simulink model "lazo_cerrado"  (Simulink 7.6)
settings: Solver=ode45  StartTime=0.0  StopTime=10.0  RelTol=1e-3
values from neighbouring files (symbols this model uses):
  K = [-0.22360679775 6.24198343522e-16 0.22360679775 -2.24770339741e-15 0 0 0 0 4.72115563111e-31 -4.72115563111e-31 4.72115563111e-31 -4.72115563111e-31 ... (144 elements, 12x12)]    [K.mat]
undefined symbols (not defined in the file or in its folder): g, Ixx, Iyy, Izz, Izzm, L, M, phi0, psi0, theta0, vq10, vq20, vq30, wq10, wq20, wq30, x0, y0, z0
settings Model: Creator=pater  LastModifiedBy=pater

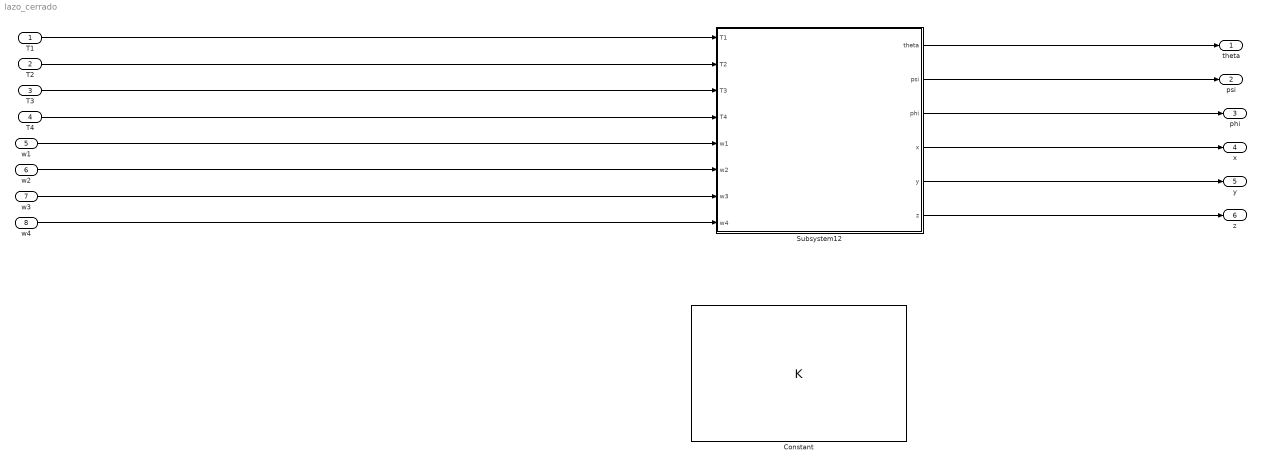
== system lazo_cerrado ==
  T1 : Inport
  T2 : Inport  Port=2
  T3 : Inport  Port=3
  T4 : Inport  Port=4
  w1 : Inport  Port=5
  w2 : Inport  Port=6
  w3 : Inport  Port=7
  w4 : Inport  Port=8
  Constant : Constant  Value=K
  Subsystem12 : Subsystem
  theta : Outport
  psi : Outport  Port=2
  phi : Outport  Port=3
  x : Outport  Port=4
  y : Outport  Port=5
  z : Outport  Port=6
  wires:
  Subsystem12/1(theta) -> theta/1
  Subsystem12/2(psi) -> psi/1
  Subsystem12/3(phi) -> phi/1
  Subsystem12/4(x) -> x/1
  Subsystem12/5(y) -> y/1
  Subsystem12/6(z) -> z/1
  w4/1 -> Subsystem12/8(w4)
  w3/1 -> Subsystem12/7(w3)
  w2/1 -> Subsystem12/6(w2)
  w1/1 -> Subsystem12/5(w1)
  T4/1 -> Subsystem12/4(T4)
  T3/1 -> Subsystem12/3(T3)
  T2/1 -> Subsystem12/2(T2)
  T1/1 -> Subsystem12/1(T1)

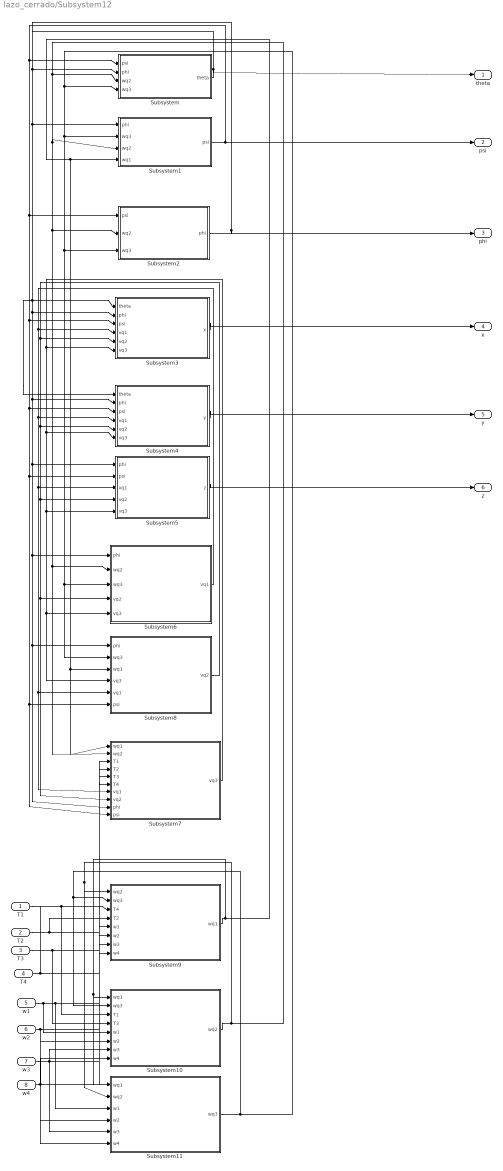
== system lazo_cerrado/Subsystem12 ==
  T1 : Inport
  T2 : Inport  Port=2
  T3 : Inport  Port=3
  T4 : Inport  Port=4
  w1 : Inport  Port=5
  w2 : Inport  Port=6
  w3 : Inport  Port=7
  w4 : Inport  Port=8
  Subsystem : Subsystem
  Subsystem1 : Subsystem
  Subsystem10 : Subsystem
  Subsystem11 : Subsystem
  Subsystem2 : Subsystem
  Subsystem3 : Subsystem
  Subsystem4 : Subsystem
  Subsystem5 : Subsystem
  Subsystem6 : Subsystem
  Subsystem7 : Subsystem
  Subsystem8 : Subsystem
  Subsystem9 : Subsystem
  theta : Outport
  psi : Outport  Port=2
  phi : Outport  Port=3
  x : Outport  Port=4
  y : Outport  Port=5
  z : Outport  Port=6
  wires:
  Subsystem/1(theta) -> Subsystem3/1(theta), Subsystem4/1(theta), theta/1
  Subsystem1/1(psi) -> Subsystem/1(psi), Subsystem2/1(psi), Subsystem3/3(psi), Subsystem4/3(psi), Subsystem5/2(psi), Subsystem8/6(psi), Subsystem7/10(psi), psi/1
  Subsystem2/1(phi) -> phi/1, Subsystem/2(phi), Subsystem1/1(phi), Subsystem3/2(phi), Subsystem4/2(phi), Subsystem5/1(phi), Subsystem6/1(phi), Subsystem8/1(phi), Subsystem7/9(phi)
  Subsystem5/1(z) -> z/1
  Subsystem4/1(y) -> y/1
  Subsystem3/1(x) -> x/1
  Subsystem6/1(vq1) -> Subsystem3/4(vq1), Subsystem4/4(vq1), Subsystem5/3(vq1), Subsystem8/5(vq1), Subsystem7/7(vq1)
  Subsystem8/1(vq2) -> Subsystem3/5(vq2), Subsystem4/5(vq2), Subsystem5/4(vq2), Subsystem6/4(vq2), Subsystem7/8(vq2)
  Subsystem7/1(vq3) -> Subsystem4/6(vq3), Subsystem5/5(vq3), Subsystem6/5(vq3), Subsystem8/4(vq3), Subsystem3/6(vq3)
  Subsystem9/1(wq1) -> Subsystem10/1(wq1), Subsystem11/1(wq1), Subsystem1/4(wq1), Subsystem8/3(wq1), Subsystem7/1(wq1)
  Subsystem10/1(wq2) -> Subsystem/3(wq2), Subsystem1/3(wq2), Subsystem2/2(wq2), Subsystem6/2(wq2), Subsystem7/2(wq2), Subsystem9/1(wq2), Subsystem11/2(wq2)
  Subsystem11/1(wq3) -> Subsystem/4(wq3), Subsystem1/2(wq3), Subsystem2/3(wq3), Subsystem6/3(wq3), Subsystem8/2(wq3), Subsystem9/2(wq3), Subsystem10/2(wq3)
  w1/1 -> Subsystem10/5(w1), Subsystem9/5(w1), Subsystem11/3(w1)
  w2/1 -> Subsystem9/6(w2), Subsystem10/6(w2), Subsystem11/4(w2)
  w3/1 -> Subsystem9/7(w3), Subsystem10/7(w3), Subsystem11/5(w3)
  w4/1 -> Subsystem9/8(w4), Subsystem10/8(w4), Subsystem11/6(w4)
  T1/1 -> Subsystem7/3(T1)
  T2/1 -> Subsystem7/4(T2), Subsystem9/4(T2)
  T3/1 -> Subsystem7/5(T3), Subsystem10/4(T3)
  T4/1 -> Subsystem7/6(T4), Subsystem9/3(T4), Subsystem10/3(T1)

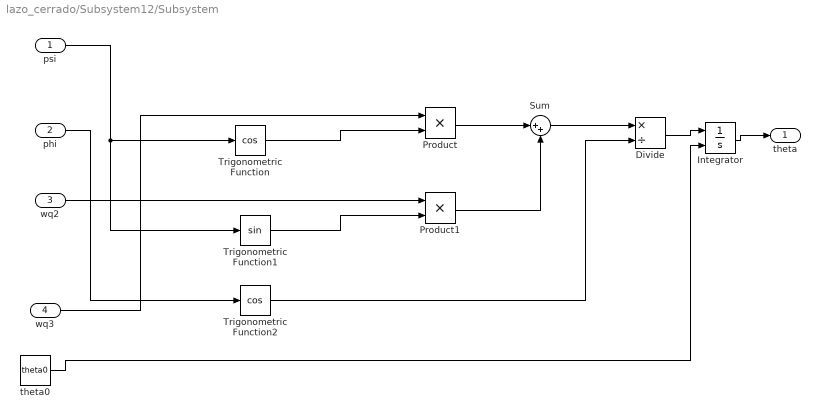
== system lazo_cerrado/Subsystem12/Subsystem ==
  psi : Inport
  phi : Inport  Port=2
  wq2 : Inport  Port=3
  wq3 : Inport  Port=4
  Divide : Product  Inputs=*/
  Integrator : Integrator  InitialConditionSource=external
  Product : Product  RndMeth=Zero
  Product1 : Product  RndMeth=Zero
  Sum : Sum  Inputs=|++
  Trigonometric Function : Trigonometry  Operator=cos
  Trigonometric Function1 : Trigonometry
  Trigonometric Function2 : Trigonometry  Operator=cos
  theta0 : Constant  Value=theta0
  theta : Outport
  wires:
  wq3/1 -> Product/1
  wq2/1 -> Product1/1
  Product/1 -> Sum/1
  Product1/1 -> Sum/2
  Sum/1 -> Divide/1
  Trigonometric Function2/1 -> Divide/2
  Divide/1 -> Integrator/1
  Trigonometric Function/1 -> Product/2
  Trigonometric Function1/1 -> Product1/2
  phi/1 -> Trigonometric Function2/1
  Integrator/1 -> theta/1
  psi/1 -> Trigonometric Function/1, Trigonometric Function1/1
  theta0/1 -> Integrator/2

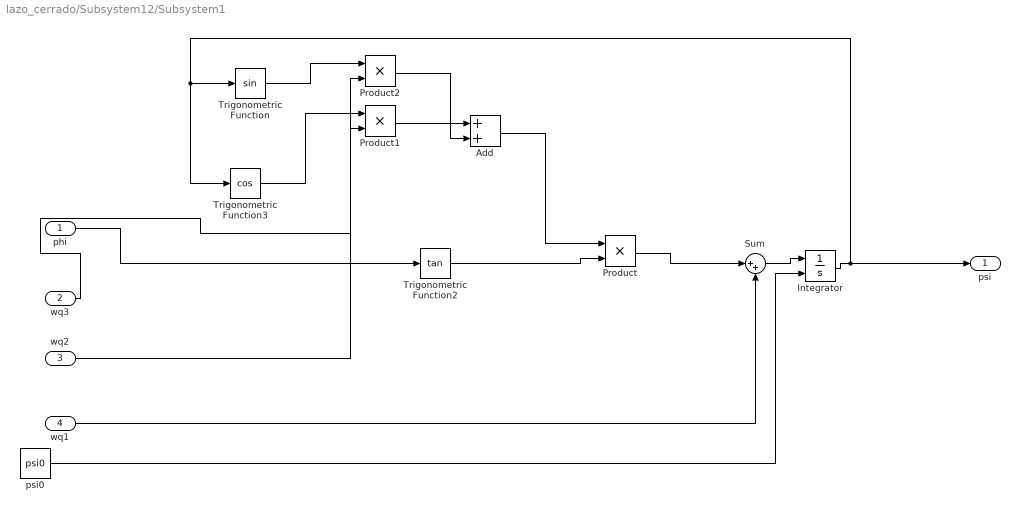
== system lazo_cerrado/Subsystem12/Subsystem1 ==
  phi : Inport
  wq3 : Inport  Port=2
  wq2 : Inport  Port=3
  wq1 : Inport  Port=4
  Add : Sum
  Integrator : Integrator  InitialConditionSource=external
  Product : Product  RndMeth=Zero
  Product1 : Product  RndMeth=Zero
  Product2 : Product  RndMeth=Zero
  Sum : Sum  Inputs=|++
  Trigonometric Function : Trigonometry
  Trigonometric Function2 : Trigonometry  Operator=tan
  Trigonometric Function3 : Trigonometry  Operator=cos
  psi0 : Constant  Value=psi0
  psi : Outport
  wires:
  Integrator/1 -> psi/1, Trigonometric Function3/1, Trigonometric Function/1
  Product/1 -> Sum/1
  phi/1 -> Trigonometric Function2/1
  Trigonometric Function2/1 -> Product/2
  wq3/1 -> Product1/2
  Trigonometric Function3/1 -> Product1/1
  Product1/1 -> Add/1
  Add/1 -> Product/1
  Trigonometric Function/1 -> Product2/1
  wq2/1 -> Product2/2
  Product2/1 -> Add/2
  wq1/1 -> Sum/2
  Sum/1 -> Integrator/1
  psi0/1 -> Integrator/2

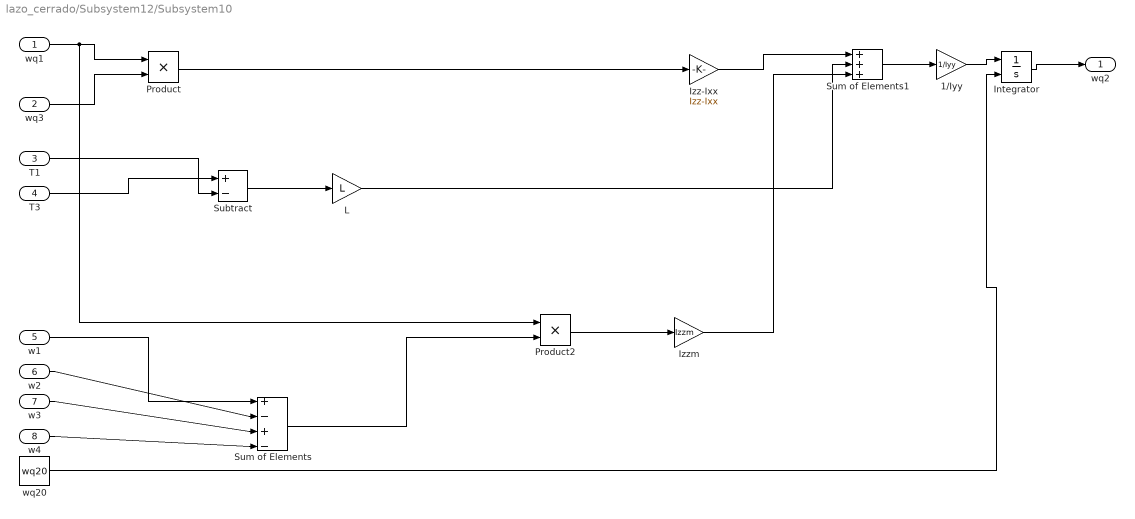
== system lazo_cerrado/Subsystem12/Subsystem10 ==
  wq1 : Inport
  wq3 : Inport  Port=2
  T1 : Inport  Port=3
  T3 : Inport  Port=4
  w1 : Inport  Port=5
  w2 : Inport  Port=6
  w3 : Inport  Port=7
  w4 : Inport  Port=8
  1/Iyy : Gain  Gain=1/Iyy
  Integrator : Integrator  InitialConditionSource=external
  Izz-Ixx : Gain  Gain=Izz-Ixx
  Izzm : Gain  Gain=Izzm
  L : Gain  Gain=L
  Product : Product  RndMeth=Zero
  Product2 : Product  RndMeth=Zero
  Subtract : Sum  Inputs=+-
  Sum of Elements : Sum  Inputs=+|-|+|-|
  Sum of Elements1 : Sum  Inputs=3
  wq20 : Constant  Value=wq20
  wq2 : Outport
  wires:
  wq1/1 -> Product/1, Product2/1
  wq3/1 -> Product/2
  Product/1 -> Izz-Ixx/1
  T3/1 -> Subtract/1
  T1/1 -> Subtract/2
  w1/1 -> Sum of Elements/1
  w2/1 -> Sum of Elements/2
  w3/1 -> Sum of Elements/3
  w4/1 -> Sum of Elements/4
  Sum of Elements/1 -> Product2/2
  Product2/1 -> Izzm/1
  Izzm/1 -> Sum of Elements1/3
  Sum of Elements1/1 -> 1/Iyy/1
  1/Iyy/1 -> Integrator/1
  Integrator/1 -> wq2/1
  Subtract/1 -> L/1
  Izz-Ixx/1 -> Sum of Elements1/1
  L/1 -> Sum of Elements1/2
  wq20/1 -> Integrator/2

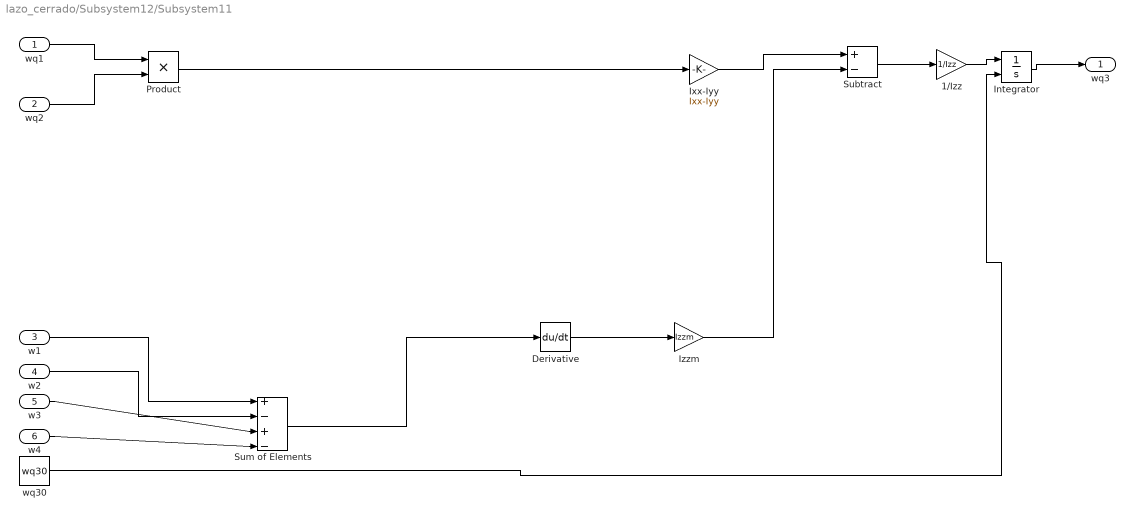
== system lazo_cerrado/Subsystem12/Subsystem11 ==
  wq1 : Inport
  wq2 : Inport  Port=2
  w1 : Inport  Port=3
  w2 : Inport  Port=4
  w3 : Inport  Port=5
  w4 : Inport  Port=6
  1/Izz : Gain  Gain=1/Izz
  Derivative : Derivative
  Integrator : Integrator  InitialConditionSource=external
  Ixx-Iyy : Gain  Gain=Ixx-Iyy
  Izzm : Gain  Gain=Izzm
  Product : Product  RndMeth=Zero
  Subtract : Sum  Inputs=+-
  Sum of Elements : Sum  Inputs=+|-|+|-|
  wq30 : Constant  Value=wq30
  wq3 : Outport
  wires:
  wq1/1 -> Product/1
  wq2/1 -> Product/2
  Product/1 -> Ixx-Iyy/1
  w1/1 -> Sum of Elements/1
  w2/1 -> Sum of Elements/2
  w3/1 -> Sum of Elements/3
  w4/1 -> Sum of Elements/4
  Sum of Elements/1 -> Derivative/1
  Derivative/1 -> Izzm/1
  Izzm/1 -> Subtract/2
  Subtract/1 -> 1/Izz/1
  1/Izz/1 -> Integrator/1
  Integrator/1 -> wq3/1
  Ixx-Iyy/1 -> Subtract/1
  wq30/1 -> Integrator/2

== system lazo_cerrado/Subsystem12/Subsystem2 ==
  psi : Inport
  wq2 : Inport  Port=2
  wq3 : Inport  Port=3
  Integrator : Integrator  InitialConditionSource=external
  Product : Product  RndMeth=Zero
  Product1 : Product  RndMeth=Zero
  Subtract : Sum  Inputs=+-
  Trigonometric Function : Trigonometry  Operator=cos
  Trigonometric Function1 : Trigonometry
  phi0 : Constant  Value=phi0
  phi : Outport
  wires:
  Integrator/1 -> phi/1
  Subtract/1 -> Integrator/1
  Product/1 -> Subtract/1
  Product1/1 -> Subtract/2
  Trigonometric Function/1 -> Product/1
  psi/1 -> Trigonometric Function/1, Trigonometric Function1/1
  Trigonometric Function1/1 -> Product1/1
  wq2/1 -> Product/2
  wq3/1 -> Product1/2
  phi0/1 -> Integrator/2

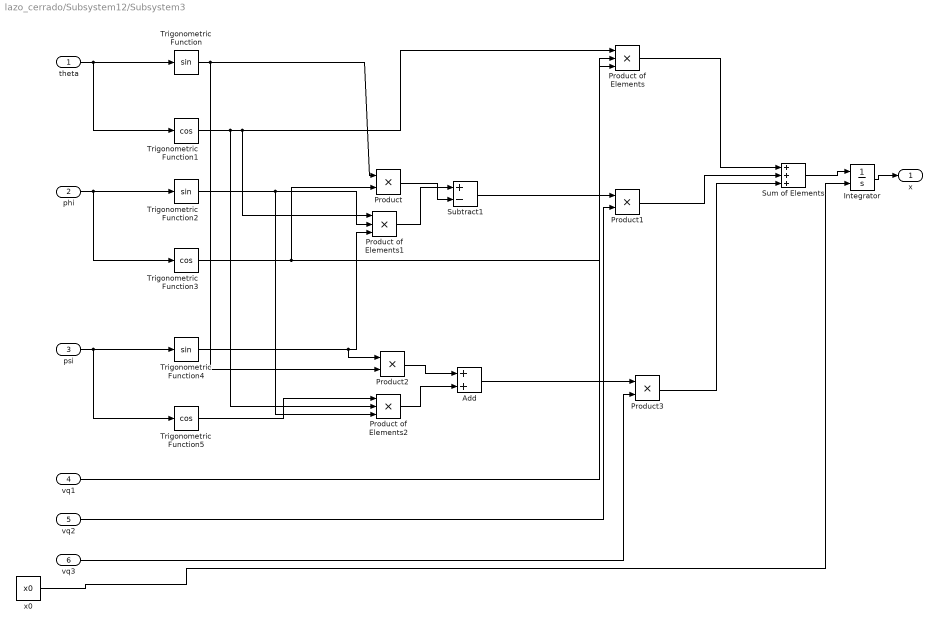
== system lazo_cerrado/Subsystem12/Subsystem3 ==
  theta : Inport
  phi : Inport  Port=2
  psi : Inport  Port=3
  vq1 : Inport  Port=4
  vq2 : Inport  Port=5
  vq3 : Inport  Port=6
  Add : Sum
  Integrator : Integrator  InitialConditionSource=external
  Product{,1..3} (4 alike) : Product  RndMeth=Zero
  Product of Elements : Product  Inputs=3
  Product of Elements1 : Product  Inputs=3
  Product of Elements2 : Product  Inputs=3
  Subtract1 : Sum  Inputs=+-
  Sum of Elements : Sum  Inputs=3
  Trigonometric Function : Trigonometry
  Trigonometric Function1 : Trigonometry  Operator=cos
  Trigonometric Function2 : Trigonometry
  Trigonometric Function3 : Trigonometry  Operator=cos
  Trigonometric Function4 : Trigonometry
  Trigonometric Function5 : Trigonometry  Operator=cos
  x0 : Constant  Value=x0
  x : Outport
  wires:
  theta/1 -> Trigonometric Function/1, Trigonometric Function1/1
  phi/1 -> Trigonometric Function2/1, Trigonometric Function3/1
  psi/1 -> Trigonometric Function4/1, Trigonometric Function5/1
  Trigonometric Function1/1 -> Product of Elements/1, Product of Elements1/1, Product of Elements2/2
  Trigonometric Function3/1 -> Product of Elements/2, Product/2
  vq1/1 -> Product of Elements/3
  Trigonometric Function/1 -> Product/1, Product2/2
  Trigonometric Function2/1 -> Product of Elements1/2, Product of Elements2/3
  Trigonometric Function4/1 -> Product of Elements1/3, Product2/1
  Subtract1/1 -> Product1/1
  vq2/1 -> Product1/2
  Product2/1 -> Add/1
  Product of Elements2/1 -> Add/2
  Trigonometric Function5/1 -> Product of Elements2/1
  Add/1 -> Product3/1
  vq3/1 -> Product3/2
  Product of Elements/1 -> Sum of Elements/1
  Product1/1 -> Sum of Elements/2
  Product3/1 -> Sum of Elements/3
  Sum of Elements/1 -> Integrator/1
  Integrator/1 -> x/1
  Product of Elements1/1 -> Subtract1/1
  Product/1 -> Subtract1/2
  x0/1 -> Integrator/2

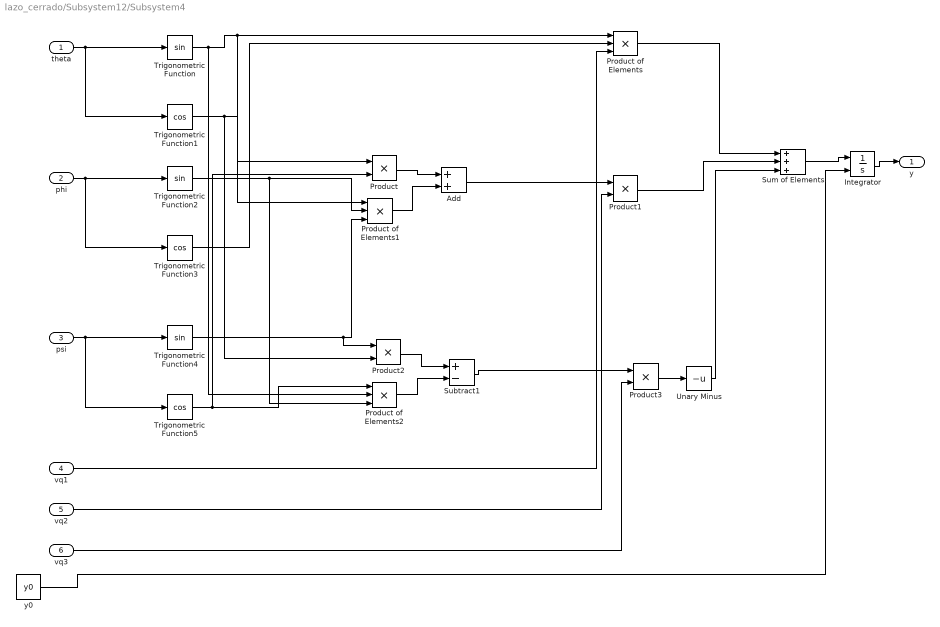
== system lazo_cerrado/Subsystem12/Subsystem4 ==
  theta : Inport
  phi : Inport  Port=2
  psi : Inport  Port=3
  vq1 : Inport  Port=4
  vq2 : Inport  Port=5
  vq3 : Inport  Port=6
  Add : Sum
  Integrator : Integrator  InitialConditionSource=external
  Product{,1..3} (4 alike) : Product  RndMeth=Zero
  Product of Elements : Product  Inputs=3
  Product of Elements1 : Product  Inputs=3
  Product of Elements2 : Product  Inputs=3
  Subtract1 : Sum  Inputs=+-
  Sum of Elements : Sum  Inputs=3
  Trigonometric Function : Trigonometry
  Trigonometric Function1 : Trigonometry  Operator=cos
  Trigonometric Function2 : Trigonometry
  Trigonometric Function3 : Trigonometry  Operator=cos
  Trigonometric Function4 : Trigonometry
  Trigonometric Function5 : Trigonometry  Operator=cos
  Unary Minus : UnaryMinus
  y0 : Constant  Value=y0
  y : Outport
  wires:
  theta/1 -> Trigonometric Function/1, Trigonometric Function1/1
  phi/1 -> Trigonometric Function2/1, Trigonometric Function3/1
  psi/1 -> Trigonometric Function4/1, Trigonometric Function5/1
  Trigonometric Function1/1 -> Product/1, Product2/2
  Trigonometric Function3/1 -> Product of Elements/2
  vq1/1 -> Product of Elements/3
  Trigonometric Function/1 -> Product of Elements/1, Product of Elements1/1, Product of Elements2/2
  Trigonometric Function2/1 -> Product of Elements1/2, Product of Elements2/3
  Trigonometric Function4/1 -> Product of Elements1/3, Product2/1
  Product/1 -> Add/1
  Product of Elements1/1 -> Add/2
  Add/1 -> Product1/1
  vq2/1 -> Product1/2
  Trigonometric Function5/1 -> Product of Elements2/1, Product/2
  Subtract1/1 -> Product3/1
  vq3/1 -> Product3/2
  Product of Elements/1 -> Sum of Elements/1
  Product1/1 -> Sum of Elements/2
  Product3/1 -> Unary Minus/1
  Sum of Elements/1 -> Integrator/1
  Integrator/1 -> y/1
  Unary Minus/1 -> Sum of Elements/3
  Product of Elements2/1 -> Subtract1/2
  Product2/1 -> Subtract1/1
  y0/1 -> Integrator/2

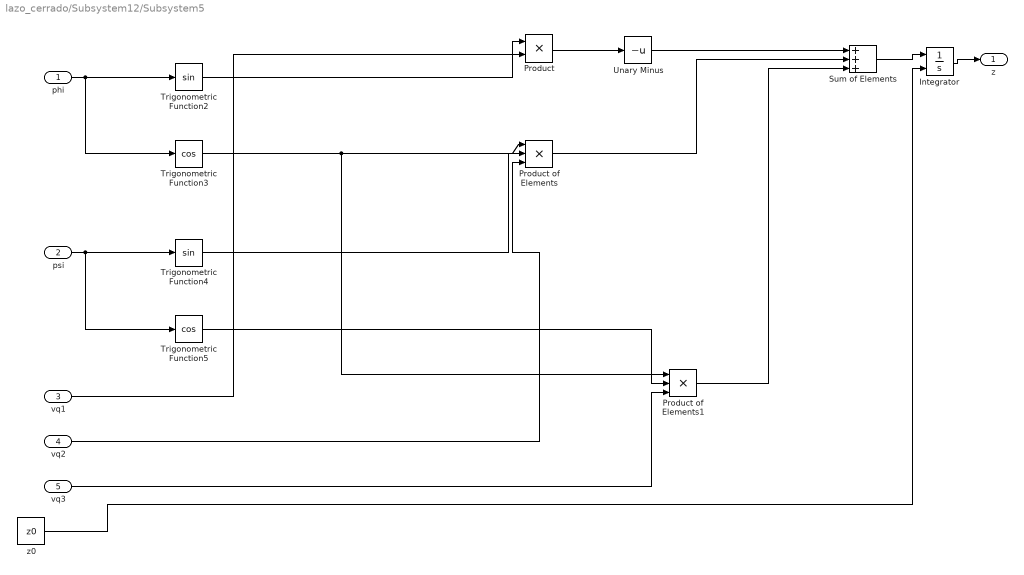
== system lazo_cerrado/Subsystem12/Subsystem5 ==
  phi : Inport
  psi : Inport  Port=2
  vq1 : Inport  Port=3
  vq2 : Inport  Port=4
  vq3 : Inport  Port=5
  Integrator : Integrator  InitialConditionSource=external
  Product : Product  RndMeth=Zero
  Product of Elements : Product  Inputs=3
  Product of Elements1 : Product  Inputs=3
  Sum of Elements : Sum  Inputs=3
  Trigonometric Function2 : Trigonometry
  Trigonometric Function3 : Trigonometry  Operator=cos
  Trigonometric Function4 : Trigonometry
  Trigonometric Function5 : Trigonometry  Operator=cos
  Unary Minus : UnaryMinus
  z0 : Constant  Value=z0
  z : Outport
  wires:
  phi/1 -> Trigonometric Function2/1, Trigonometric Function3/1
  psi/1 -> Trigonometric Function4/1, Trigonometric Function5/1
  Sum of Elements/1 -> Integrator/1
  Integrator/1 -> z/1
  Trigonometric Function2/1 -> Product/1
  vq1/1 -> Product/2
  Product/1 -> Unary Minus/1
  Trigonometric Function3/1 -> Product of Elements/1, Product of Elements1/1
  Trigonometric Function4/1 -> Product of Elements/2
  vq2/1 -> Product of Elements/3
  Trigonometric Function5/1 -> Product of Elements1/2
  vq3/1 -> Product of Elements1/3
  Product of Elements/1 -> Sum of Elements/2
  Product of Elements1/1 -> Sum of Elements/3
  Unary Minus/1 -> Sum of Elements/1
  z0/1 -> Integrator/2

== system lazo_cerrado/Subsystem12/Subsystem6 ==
  phi : Inport
  wq2 : Inport  Port=2
  wq3 : Inport  Port=3
  vq2 : Inport  Port=4
  vq3 : Inport  Port=5
  Add : Sum
  Integrator : Integrator  InitialConditionSource=external
  Product : Product  RndMeth=Zero
  Product1 : Product  RndMeth=Zero
  Subtract : Sum  Inputs=+-
  Trigonometric Function4 : Trigonometry
  gravedad : Gain  Gain=-g
  vq10 : Constant  Value=vq10
  vq1 : Outport
  wires:
  phi/1 -> Trigonometric Function4/1
  vq2/1 -> Product/2
  wq3/1 -> Product/1
  vq3/1 -> Product1/2
  wq2/1 -> Product1/1
  Product/1 -> Subtract/1
  Product1/1 -> Subtract/2
  Trigonometric Function4/1 -> gravedad/1
  gravedad/1 -> Add/1
  Subtract/1 -> Add/2
  Add/1 -> Integrator/1
  Integrator/1 -> vq1/1
  vq10/1 -> Integrator/2

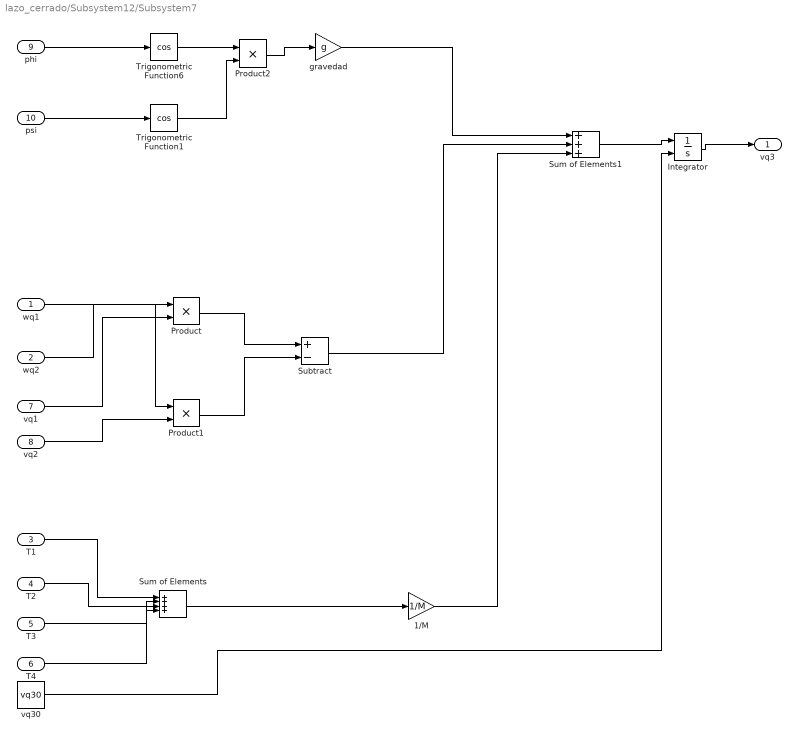
== system lazo_cerrado/Subsystem12/Subsystem7 ==
  wq1 : Inport
  wq2 : Inport  Port=2
  T1 : Inport  Port=3
  T2 : Inport  Port=4
  T3 : Inport  Port=5
  T4 : Inport  Port=6
  vq1 : Inport  Port=7
  vq2 : Inport  Port=8
  phi : Inport  Port=9
  psi : Inport  Port=10
  1/M : Gain  Gain=1/M
  Integrator : Integrator  InitialConditionSource=external
  Product : Product  RndMeth=Zero
  Product1 : Product  RndMeth=Zero
  Product2 : Product  RndMeth=Zero
  Subtract : Sum  Inputs=+-
  Sum of Elements : Sum  Inputs=4
  Sum of Elements1 : Sum  Inputs=3
  Trigonometric Function1 : Trigonometry  Operator=cos
  Trigonometric Function6 : Trigonometry  Operator=cos
  gravedad : Gain  Gain=g
  vq30 : Constant  Value=vq30
  vq3 : Outport
  wires:
  T1/1 -> Sum of Elements/1
  T2/1 -> Sum of Elements/2
  T3/1 -> Sum of Elements/3
  T4/1 -> Sum of Elements/4
  Sum of Elements/1 -> 1/M/1
  vq1/1 -> Product/2
  wq2/1 -> Product/1
  vq2/1 -> Product1/2
  wq1/1 -> Product1/1
  Product/1 -> Subtract/1
  Product1/1 -> Subtract/2
  phi/1 -> Trigonometric Function6/1
  psi/1 -> Trigonometric Function1/1
  Trigonometric Function1/1 -> Product2/2
  gravedad/1 -> Sum of Elements1/1
  Subtract/1 -> Sum of Elements1/2
  1/M/1 -> Sum of Elements1/3
  Sum of Elements1/1 -> Integrator/1
  Integrator/1 -> vq3/1
  Trigonometric Function6/1 -> Product2/1
  Product2/1 -> gravedad/1
  vq30/1 -> Integrator/2

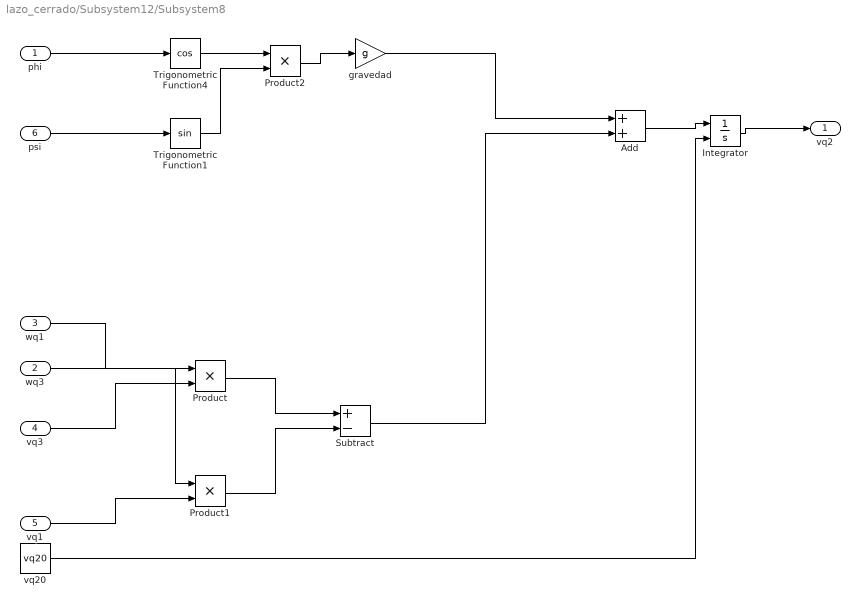
== system lazo_cerrado/Subsystem12/Subsystem8 ==
  phi : Inport
  wq3 : Inport  Port=2
  wq1 : Inport  Port=3
  vq3 : Inport  Port=4
  vq1 : Inport  Port=5
  psi : Inport  Port=6
  Add : Sum
  Integrator : Integrator  InitialConditionSource=external
  Product : Product  RndMeth=Zero
  Product1 : Product  RndMeth=Zero
  Product2 : Product  RndMeth=Zero
  Subtract : Sum  Inputs=+-
  Trigonometric Function1 : Trigonometry
  Trigonometric Function4 : Trigonometry  Operator=cos
  gravedad : Gain  Gain=g
  vq20 : Constant  Value=vq20
  vq2 : Outport
  wires:
  phi/1 -> Trigonometric Function4/1
  vq3/1 -> Product/2
  wq1/1 -> Product/1
  vq1/1 -> Product1/2
  wq3/1 -> Product1/1
  Product/1 -> Subtract/1
  Product1/1 -> Subtract/2
  gravedad/1 -> Add/1
  Subtract/1 -> Add/2
  Add/1 -> Integrator/1
  Integrator/1 -> vq2/1
  psi/1 -> Trigonometric Function1/1
  Trigonometric Function1/1 -> Product2/2
  Trigonometric Function4/1 -> Product2/1
  Product2/1 -> gravedad/1
  vq20/1 -> Integrator/2

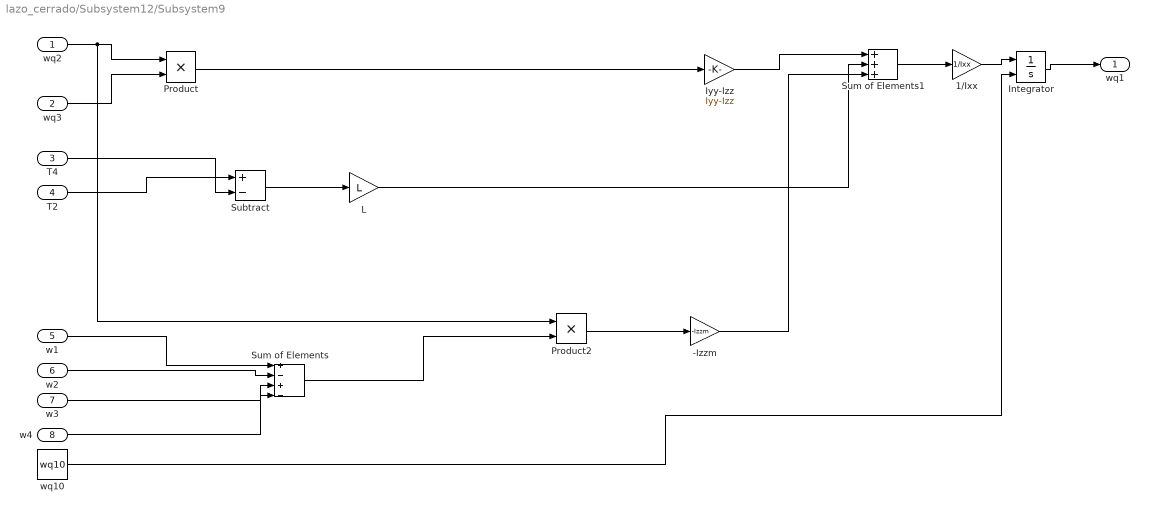
== system lazo_cerrado/Subsystem12/Subsystem9 ==
  wq2 : Inport
  wq3 : Inport  Port=2
  T4 : Inport  Port=3
  T2 : Inport  Port=4
  w1 : Inport  Port=5
  w2 : Inport  Port=6
  w3 : Inport  Port=7
  w4 : Inport  Port=8
  -Izzm : Gain  Gain=-Izzm
  1/Ixx : Gain  Gain=1/Ixx
  Integrator : Integrator  InitialConditionSource=external
  Iyy-Izz : Gain  Gain=Iyy-Izz
  L : Gain  Gain=L
  Product : Product  RndMeth=Zero
  Product2 : Product  RndMeth=Zero
  Subtract : Sum  Inputs=+-
  Sum of Elements : Sum  Inputs=+|-|+|-
  Sum of Elements1 : Sum  Inputs=3
  wq10 : Constant  Value=wq10
  wq1 : Outport
  wires:
  wq2/1 -> Product/1, Product2/1
  wq3/1 -> Product/2
  Product/1 -> Iyy-Izz/1
  T2/1 -> Subtract/1
  T4/1 -> Subtract/2
  w1/1 -> Sum of Elements/1
  w3/1 -> Sum of Elements/3
  w4/1 -> Sum of Elements/4
  Sum of Elements/1 -> Product2/2
  Product2/1 -> -Izzm/1
  -Izzm/1 -> Sum of Elements1/3
  Sum of Elements1/1 -> 1/Ixx/1
  1/Ixx/1 -> Integrator/1
  Integrator/1 -> wq1/1
  Subtract/1 -> L/1
  Iyy-Izz/1 -> Sum of Elements1/1
  L/1 -> Sum of Elements1/2
  w2/1 -> Sum of Elements/2
  wq10/1 -> Integrator/2
